simulink model "hw2_model"  (R2016a)
settings: Solver=VariableStepAuto  StartTime=0.0  StopTime=0.2  MinStep=1e-6  RelTol=1e-6
values from neighbouring files (symbols this model uses):
  wr = 100    [hw2.m]
settings Model: Creator=Seth Barger  LastModifiedBy=Seth Barger

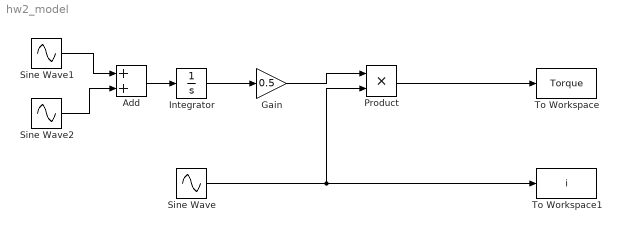
== system hw2_model ==
  Add : Sum
  Gain : Gain  Gain=0.5
  Integrator : Integrator
  Product : Product
  Sine Wave : Sin  Amplitude=5  Frequency=wr  Samples=100  SampleTime=0
  Sine Wave1 : Sin  Amplitude=.015  Frequency=wr  Phase=pi/2  Samples=100  SampleTime=0
  Sine Wave2 : Sin  Amplitude=.03  Frequency=3*wr  Phase=pi/2  Samples=100  SampleTime=0
  To Workspace : ToWorkspace  VariableName=Torque  SaveFormat=Timeseries  SampleTime=-1
  To Workspace1 : ToWorkspace  VariableName=i  SaveFormat=Timeseries  SampleTime=-1
  wires:
  Sine Wave/1 -> Product/2, To Workspace1/1
  Integrator/1 -> Gain/1
  Gain/1 -> Product/1
  Product/1 -> To Workspace/1
  Add/1 -> Integrator/1
  Sine Wave1/1 -> Add/1
  Sine Wave2/1 -> Add/2
